simulink model "CSD_final"  (R2018b)
settings: Solver=VariableStepAuto  StartTime=0.0  StopTime=10.0  RelTol=1e-3
settings Model: Creator=ohsna  LastModifiedBy=ohsna
settings DebuggingCC: UnderSpecifiedDimensionMsg=warning

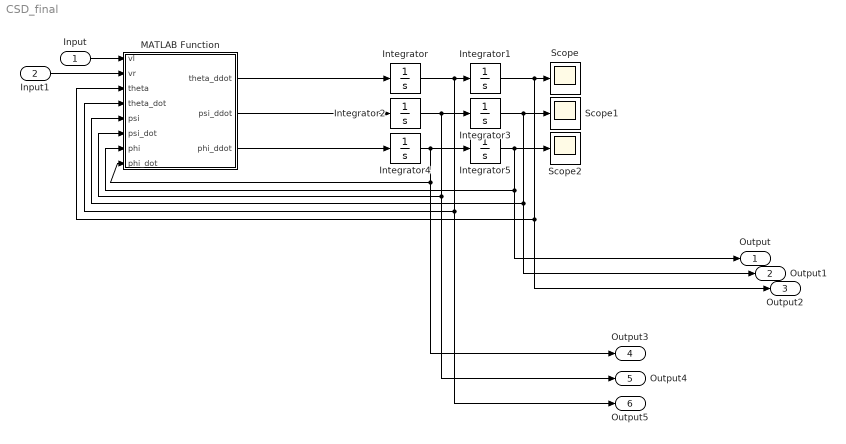
== system CSD_final ==
  Input : Inport  PortDimensions=1
  Input1 : Inport  Port=2  PortDimensions=1
  Integrator{,1..2,4..5} (5 alike) : Integrator
  Integrator3 : Integrator  InitialCondition=1
  MATLAB Function : MATLAB Function  TreatAsAtomicUnit=on
  Scope : Scope
  Scope1 : Scope
  Scope2 : Scope
  Output : Outport
  Output1 : Outport  Port=2
  Output2 : Outport  Port=3
  Output3 : Outport  Port=4
  Output4 : Outport  Port=5
  Output5 : Outport  Port=6
  wires:
  Integrator/1 -> Integrator1/1, Output5/1, MATLAB Function/4(theta_dot)
  Integrator2/1 -> Integrator3/1, Output4/1, MATLAB Function/6(psi_dot)
  Integrator4/1 -> Integrator5/1, Output3/1, MATLAB Function/8(phi_dot)
  Integrator1/1 -> Scope/1, MATLAB Function/3(theta), Output2/1
  Integrator3/1 -> Scope1/1, Output1/1, MATLAB Function/5(psi)
  Integrator5/1 -> Scope2/1, Output/1, MATLAB Function/7(phi)
  Input1/1 -> MATLAB Function/2(vr)
  Input/1 -> MATLAB Function/1(vl)
  MATLAB Function/3(phi_ddot) -> Integrator4/1
  MATLAB Function/2(psi_ddot) -> Integrator2/1
  MATLAB Function/1(theta_ddot) -> Integrator/1

== matlab function CSD_final/MATLAB Function ==
  data: vl input; theta_ddot output; vr input; theta input; theta_dot input; psi input; psi_dot input; phi input; phi_dot input; psi_ddot output; phi_ddot output
function [theta_ddot, psi_ddot, phi_ddot] = fcn(vl, vr, theta, theta_dot, psi, psi_dot, phi, phi_dot)
    % mass of robot (kg)
    M = 0.6;

    % mass of wheels (kg)
    m = 0.03;

    % distance to center of mass (m)
    L = 0.125;

    % Wheel radius (m)
    R = 0.028;

    % Body width (m)
    W = 0.126;

    % Body depth (m)
    D = 0.07;

    % Acceleration due to gravity (m/s^2)
    g = 9.81;

    % Resistance (Ohms)
    Rm = 6.83;

    % Moment of inertia of robot ( kg m^2)
    Jpsi = M *(L^2) / 3;

    % Moment of inertia of body yaw (kg m^2)
    Jphi = M * (W^2 + D^2) / 12;

    % Moment of inertia of wheels (kg m^2)
    Jomega = m * R^2 / 2;

    % Moment of inertia of DC motors (kg m^2)
    Jm = 10^(-5);

    % Torque constant (Nm/A)
    kt = 0.305;

    % EMF constant (V/(rad/s))
    kb = 0.556;

    % Friction coefficient between DC motor and body
    fm = 0.0022;

    % Friction coeff between wheel and floor
    fw = 0;

    % Gear ratio
    n = 1;

    alph = n * kt / Rm;
    bet = ((n * kt * kb) / Rm) + fm;

    m4 = m*(W^2) / 2 + Jphi + ((W^2)/ (2*R^2))* (Jomega + n^2 * Jm);

    constD = M*L*L+Jpsi+2*(n*n)*Jm;
    constA = (2*m+M)*R*R+2*Jomega+2*(n*n)*Jm;

    Fpsi = calc_Fpsi(vl, vr, theta_dot, psi_dot);
    Fphi = calc_Fphi(vl, vr, phi_dot);
    Ftheta = calc_Ftheta(vl, vr, theta_dot, psi_dot);

    varB = makeB(psi);
    varC = makeC(psi, psi_dot);
    varE = makeE(psi, phi_dot);

    theta_ddot = (constD * Ftheta - varB * Fpsi + varC * constD + varB * varE) / (constA * constD - varB * varB);
    phi_ddot = (Fphi - 2*M*L*L*psi_dot*phi_dot*sin(psi)*cos(psi)) / (m*W*W/2 + Jphi + (W*W/(2*R*R))*(Jomega+n*n*Jm)+M*L*L*(sin(psi)*sin(psi)));
    psi_ddot = (-varB*Ftheta-constA*Fpsi-varB*varC+constA*varE) / (constA*constD-varB*varB);
end
